simulink model "fs_th_true"  (R2020a)
settings: Solver=ode4  StartTime=0.0  StopTime=inf  FixedStep=0.05  RelTol=1e-3
undefined symbols (not defined in the file): Angular, Linear
libraries: robotlib x15, dspstat3 x1
settings Model: Creator=ivory  LastModifiedBy=ivory
settings OptimizationCC: EnhancedBackFolding=on  PassReuseOutputArgsAs=Individual arguments  ZeroExternalMemoryAtStartup=off  ZeroInternalMemoryAtStartup=off  MaxStackSize=64  OptimizeBlockOrder=speed  DifferentSizesBufferReuse=on  OptimizationCustomize=off  EfficientTunableParamExpr=on
settings DebuggingCC: ParameterTunabilityLossMsg=error
settings HardwareCC: ProdBitPerPointer=32  ProdBitPerSizeT=32  ProdBitPerPtrDiffT=32  ProdLargestAtomicFloat=None  ProdIntDivRoundTo=Undefined  ProdEndianess=Unspecified  ProdWordSize=32  ProdHWDeviceType=Generic->Unspecified (assume 32-bit Generic)
settings SFSimCC: MATLABDynamicMemAlloc=off
settings RTWCC: SystemTargetFile=ert.tlc  HardwareBoard=Robot Operating System (ROS)  TemplateMakefile=ert_default_tmf  GenerateReport=on  Toolchain=Catkin  IncludeHyperlinkInReport=on  LaunchReport=on  TargetLang=C++  GenerateTraceInfo=on  GenerateTraceReport=on  GenerateTraceReportSl=on  GenerateTraceReportSf=on  GenerateTraceReportEml=on
settings CodeAppCC: ForceParamTrailComments=on  IgnoreCustomStorageClasses=off  OperatorAnnotations=on  SimulinkDataObjDesc=on  SFDataObjDesc=on  InsertBlockDesc=on
settings ERTTargetCC: SupportContinuousTime=on  SupportVariableSizeSignals=on

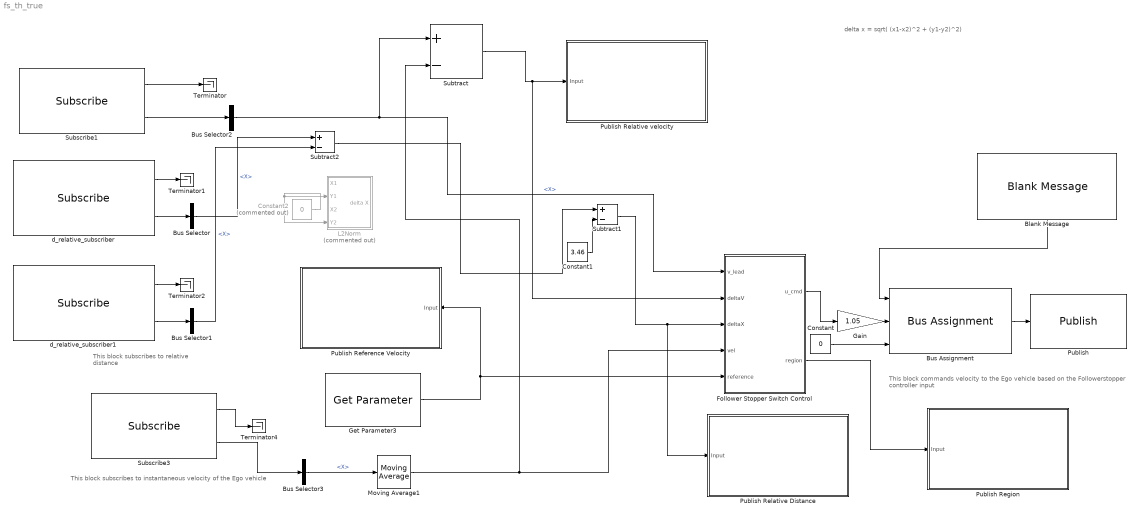
== system fs_th_true ==
  note: delta x = sqrt( (x1-x2)^2 + (y1-y2)^2)
  note: This block subscribes to
      | instantaneous velocity of the Ego vehicle
  note: This block subscribes
      | to relative distance
  note: This block commands velocity to the Ego vehicle based
      | on the Followerstopper controller input
  Blank Message : robotlib/Blank Message  messageClass=Message  entityType=geometry_msgs/Twist  messageType=geometry_msgs/Twist  SampleTime=inf
  Bus Assignment : BusAssignment  AssignedSignals=Linear.X,Angular.Z
  Bus Selector : BusSelector  OutputSignals=Pose.Pose.Position.X
  Bus Selector1 : BusSelector  OutputSignals=Pose.Pose.Position.X
  Bus Selector2 : BusSelector  OutputSignals=Linear.X
  Bus Selector3 : BusSelector  OutputSignals=Linear.X
  Constant : Constant  Value=0
  Constant1 : Constant  Value=3.46
  Constant2 : Constant  Commented=on  Value=0
  Follower Stopper Switch Control : Subsystem
  Gain : Gain  Gain=1.05
  Get Parameter3 : robotlib/Get Parameter  ParameterSource=Specify your own  ParameterName=v_ref  ParameterType=double  ParameterMaxArrayLength=16  ParameterInitialValue=4.5  SampleTime=-1  ShowErrorCodeOutput=off  ModelName=fs_th_true  BlockId=ParamGet_fs_th_true_158
      settings: SourceProductBaseCode=RR
  L2Norm : Subsystem  Commented=on
  Moving Average1 : dspstat3/Moving Average  Method=Sliding window  ForgettingFactorPort=off  SpecifyWindowLength=on  WindowLength=20  ForgettingFactor=0.9  SimulateUsing=Code generation
  Publish : robotlib/Publish  topicSource=Specify your own  topic=cmd_vel  messageType=geometry_msgs/Twist  messageQueueLength=1
  Publish Reference Velocity : Subsystem
  Publish Region : Subsystem
  Publish Relative Distance : Subsystem
  Publish Relative velocity : Subsystem
  Subscribe1 : robotlib/Subscribe  topicSource=Specify your own  topic=leadervel  messageType=geometry_msgs/Twist  sampleTime=-1  messageQueueLength=1
  Subscribe3 : robotlib/Subscribe  topicSource=Specify your own  topic=vel  messageType=geometry_msgs/Twist  sampleTime=-1  messageQueueLength=1
  Subtract : Sum  Inputs=+-
  Subtract1 : Sum  Inputs=+-
  Subtract2 : Sum  Inputs=+-
  Terminator{,1..2,4} (4 alike) : Terminator
  d_relative_subscriber : robotlib/Subscribe  topicSource=Specify your own  topic=leaderpos  messageType=nav_msgs/Odometry  sampleTime=-1  messageQueueLength=1
  d_relative_subscriber1 : robotlib/Subscribe  topicSource=Specify your own  topic=egopos  messageType=nav_msgs/Odometry  sampleTime=-1  messageQueueLength=1
  wires:
  Bus Assignment/1 -> Publish/1
  d_relative_subscriber/2 -> Bus Selector/1
  Subscribe3/2 -> Bus Selector3/1
  Blank Message/1 -> Bus Assignment/1
  Bus Selector3/1 -> Moving Average1/1  "<X>"
  Constant/1 -> Bus Assignment/3
  Subscribe3/1 -> Terminator4/1
  Follower Stopper Switch Control/1(u_cmd) -> Gain/1
  Gain/1 -> Bus Assignment/2
  d_relative_subscriber/1 -> Terminator1/1
  Moving Average1/1 -> Subtract/2, Follower Stopper Switch Control/4(vel)
  Get Parameter3/1 -> Follower Stopper Switch Control/5(reference), Publish Reference Velocity/1(Input)
  Follower Stopper Switch Control/2(region) -> Publish Region/1(Input)
  Subscribe1/1 -> Terminator/1
  d_relative_subscriber1/1 -> Terminator2/1
  d_relative_subscriber1/2 -> Bus Selector1/1
  Subscribe1/2 -> Bus Selector2/1
  Bus Selector2/1 -> Subtract/1, Follower Stopper Switch Control/1(v_lead)  "<X>"
  Subtract/1 -> Follower Stopper Switch Control/2(deltaV), Publish Relative velocity/1(Input)
  Bus Selector/1 -> Subtract2/1  "<X>"
  Bus Selector1/1 -> Subtract2/2  "<X>"
  Subtract2/1 -> Subtract1/1
  Constant1/1 -> Subtract1/2
  Subtract1/1 -> Publish Relative Distance/1(Input), Follower Stopper Switch Control/3(deltaX)
  Constant2/1 -> L2Norm/4(Y2), L2Norm/2(Y1)

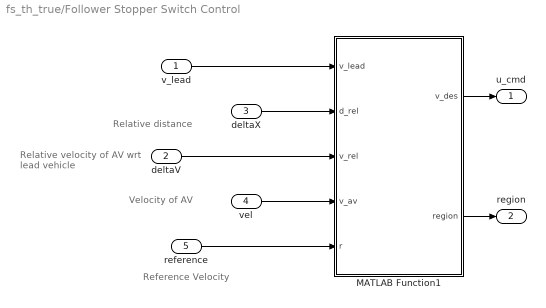
== system fs_th_true/Follower Stopper Switch Control ==
  note: Relative velocity of
      | AV wrt lead vehicle
  note: Velocity of AV
  note: Reference Velocity
  note: Relative distance
  v_lead : Inport
  deltaV : Inport  Port=2
  deltaX : Inport  Port=3
  vel : Inport  Port=4
  reference : Inport  Port=5
  MATLAB Function1 : MATLAB Function  TreatAsAtomicUnit=on
  u_cmd : Outport
  region : Outport  Port=2
  wires:
  deltaX/1 -> MATLAB Function1/2(d_rel)
  deltaV/1 -> MATLAB Function1/3(v_rel)
  vel/1 -> MATLAB Function1/4(v_av)
  v_lead/1 -> MATLAB Function1/1(v_lead)
  reference/1 -> MATLAB Function1/5(r)
  MATLAB Function1/1(v_des) -> u_cmd/1
  MATLAB Function1/2(region) -> region/1

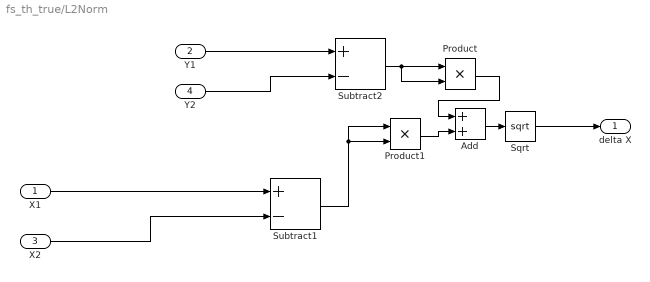
== system fs_th_true/L2Norm ==
  X1 : Inport
  Y1 : Inport  Port=2
  X2 : Inport  Port=3
  Y2 : Inport  Port=4
  Add : Sum
  Product : Product
  Product1 : Product
  Sqrt : Sqrt  SaturateOnIntegerOverflow=on
  Subtract1 : Sum  Inputs=+-
  Subtract2 : Sum  Inputs=+-
  delta X : Outport
  wires:
  Add/1 -> Sqrt/1
  Product1/1 -> Add/2
  Y1/1 -> Subtract2/1
  Sqrt/1 -> delta X/1
  Product/1 -> Add/1
  X2/1 -> Subtract1/2
  X1/1 -> Subtract1/1
  Subtract2/1 -> Product/2, Product/1
  Subtract1/1 -> Product1/2, Product1/1
  Y2/1 -> Subtract2/2

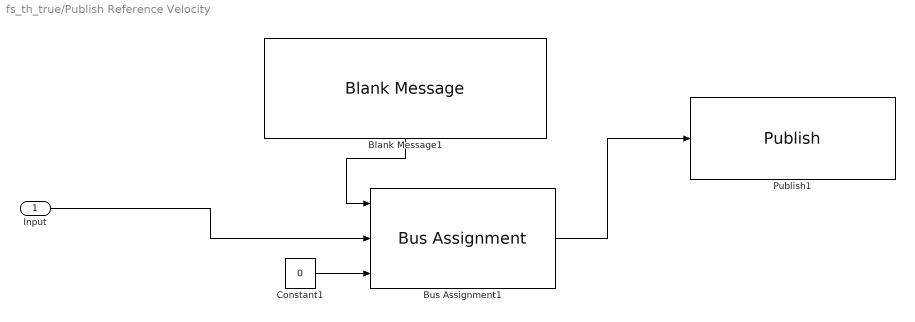
== system fs_th_true/Publish Reference Velocity ==
  Input : Inport
  Blank Message1 : robotlib/Blank Message  messageClass=Message  entityType=geometry_msgs/Twist  messageType=geometry_msgs/Twist  SampleTime=inf
  Bus Assignment1 : BusAssignment  AssignedSignals=Linear.X,Angular.Z
  Constant1 : Constant  Value=0
  Publish1 : robotlib/Publish  topicSource=Specify your own  topic=velocity_ref  messageType=geometry_msgs/Twist  messageQueueLength=1
  wires:
  Input/1 -> Bus Assignment1/2
  Constant1/1 -> Bus Assignment1/3
  Blank Message1/1 -> Bus Assignment1/1
  Bus Assignment1/1 -> Publish1/1

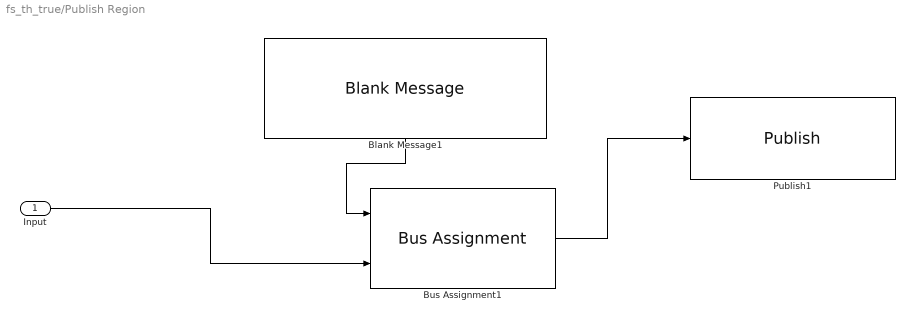
== system fs_th_true/Publish Region ==
  Input : Inport
  Blank Message1 : robotlib/Blank Message  messageClass=Message  entityType=std_msgs/UInt8  messageType=std_msgs/UInt8  SampleTime=inf
  Bus Assignment1 : BusAssignment  AssignedSignals=Data
  Publish1 : robotlib/Publish  topicSource=Specify your own  topic=region  messageType=std_msgs/UInt8  messageQueueLength=1
  wires:
  Input/1 -> Bus Assignment1/2
  Blank Message1/1 -> Bus Assignment1/1
  Bus Assignment1/1 -> Publish1/1

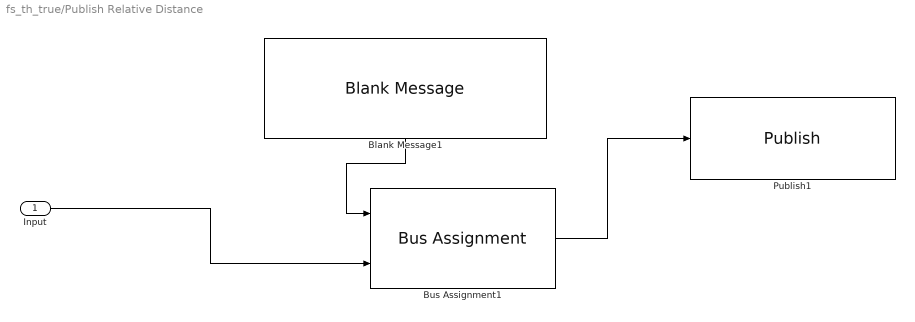
== system fs_th_true/Publish Relative Distance ==
  Input : Inport
  Blank Message1 : robotlib/Blank Message  messageClass=Message  entityType=std_msgs/Float64  messageType=std_msgs/Float64  SampleTime=inf
  Bus Assignment1 : BusAssignment  AssignedSignals=Data
  Publish1 : robotlib/Publish  topicSource=Specify your own  topic=distance_measured  messageType=std_msgs/Float64  messageQueueLength=1
  wires:
  Input/1 -> Bus Assignment1/2
  Blank Message1/1 -> Bus Assignment1/1
  Bus Assignment1/1 -> Publish1/1

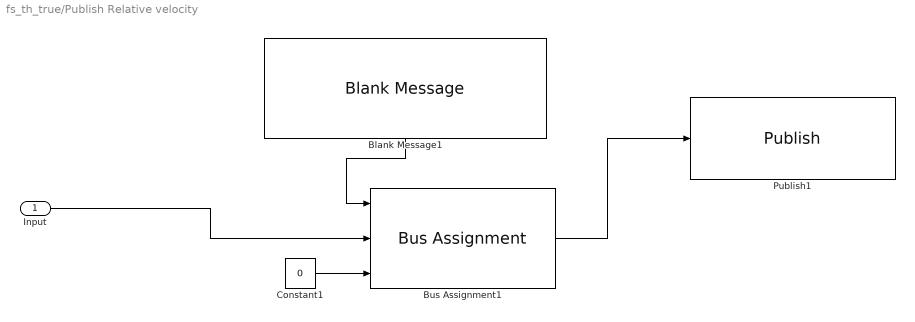
== system fs_th_true/Publish Relative velocity ==
  Input : Inport
  Blank Message1 : robotlib/Blank Message  messageClass=Message  entityType=geometry_msgs/Twist  messageType=geometry_msgs/Twist  SampleTime=inf
  Bus Assignment1 : BusAssignment  AssignedSignals=Linear.X,Angular.Z
  Constant1 : Constant  Value=0
  Publish1 : robotlib/Publish  topicSource=Specify your own  topic=v_relative_est  messageType=geometry_msgs/Twist  messageQueueLength=1
  wires:
  Input/1 -> Bus Assignment1/2
  Constant1/1 -> Bus Assignment1/3
  Blank Message1/1 -> Bus Assignment1/1
  Bus Assignment1/1 -> Publish1/1

== matlab function fs_th_true/Follower Stopper Switch Control/MATLAB Function1 ==
  data: v_lead input; v_des output; d_rel input; v_rel input; v_av input; r input; region output
function [v_des, region]= fcn(v_lead, d_rel,v_rel,v_av, r)
%#codegen
% Safety controller, based on quadratic bands.
% Input: r = desired velocity (from other models)
%          d_rel = estimate of gap to vehicle ahead
%          v_rel = estimate of time derivative of dx (= velocity difference)
%         v_AV = velocity of AV
%      dx_min = minimum distance
% dx_activate = distance below which controller does something
%       decel = vector of three deceleration values for parabolas
% Out:  u_cmd = actual velocity commanded (always u_cmd<=U)
%
% Controller-specific parameters

    w = zeros(3,1);
    alpha = zeros(3,1);
    w(1) = 4.5;
    alpha(1) = 1.5;
    w(3) = 6.0;
    alpha(3) = 0.5;
    w(2) = (w(1)+w(3))/2;
    alpha(2) = (alpha(1)+alpha(3))/2;
    if(nargin<4)
        r = 30;
    end
    
    %v_rel_star = min(v_rel,0)
    v_rel_star = v_rel;
    v_rel_star(v_rel >= 0) = 0;
   
    h_1 = 0.4;
    h_2 = 1.2;
    h_3 = 1.8;
    
    x1 = w(1) + (0.5*v_rel_star.^2)/alpha(1) + h_1*v_av;
    x2 = w(2) + (0.5*v_rel_star.^2)/alpha(2) + h_2*v_av;
    x3 = w(3) + (0.5*v_rel_star.^2)/alpha(3) + h_3*v_av;
    
%     v_lead = v_av+v_rel;
    
    
    %v = min([max([v_lead,0]),r]);
    v = v_lead;
    v(v_lead<0) = 0;
    
    v(v_lead>r) = r;
  
    v_des = zeros(size(d_rel)); 
    %safe region
    v_des(d_rel>x3) = r;  
    %adaptation region 1
    temp_v_des = v+(r-v).*(d_rel-x2)./(x3-x2);
    v_des(d_rel>x2 & d_rel<=x3) = temp_v_des(d_rel>x2 & d_rel<=x3);   
    %adaptation region 2
    temp_v_des = v.*(d_rel-x1)./(x2-x1);
    v_des(d_rel>x1 & d_rel<=x2) = temp_v_des(d_rel>x1 & d_rel<=x2); 
    
    if d_rel>x3
        region = uint8(0);
    elseif d_rel>x2 && d_rel<=x3
        region = uint8(1);
    elseif d_rel>x1 && d_rel<=x2
        region = uint8(2);
    else
        region = uint8(3);
    end
